simulink model "Q5_three_chart_system"  (R2024b)
settings: Solver=VariableStepAuto  StartTime=0.0  StopTime=100  RelTol=1e-3
model workspace (MAT data in the model file):
  K3 = 1
  M1 = 4
  M2 = 2
  M3 = 1
  b1 = 1
  b2 = 1
  b3 = 1
  k1 = 3
  k2 = 1
  k3 = 1
settings Model: Creator=chall  LastModifiedBy=chall

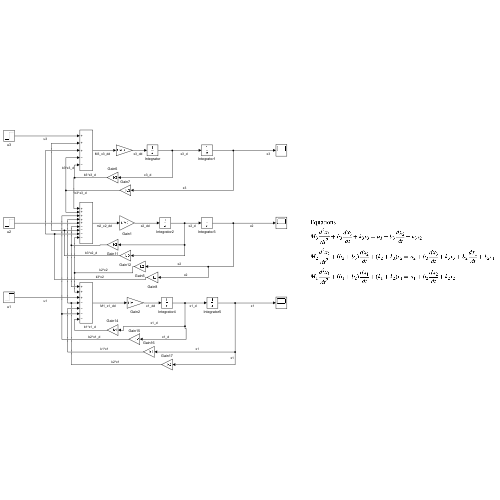
[thumbnail: Simulink's stored preview of the top-level diagram]
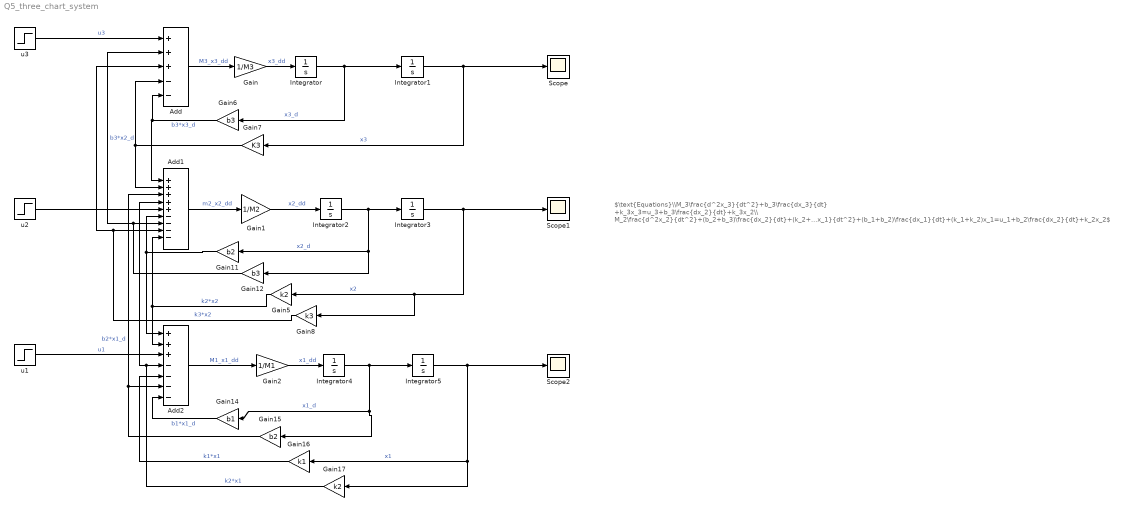
== system Q5_three_chart_system ==
  note: $\text{Equations}\\M_3\frac{d^2x_3}{dt^2}+b_3\frac{dx_3}{dt} +k_3x_3=u_3+b_3\frac{dx_2}{dt}+k_3x_2\\ M_2\frac{d^2x_2}{dt^2}+(b_2+b_3)\frac{dx_2}{dt}+(k_2+k_3)x_2=u_2+b_3\frac{dx_3}{dt}+k_3x_3+b_2\frac{dx_1}{dt}+k_2x_1\\M_1\frac{d^2x_1}{dt^2}+(b_1+b_2)\frac{dx_1}{dt}+(k_1+k_2)x_1=u_1+b_2\frac{dx_2}{dt}+k_2x_2$
  Add : Sum  Inputs=+++--
  Add1 : Sum  Inputs=+++++----
  Add2 : Sum  Inputs=+++----
  Gain : Gain  Gain=1/M3
  Gain1 : Gain  Gain=1/M2
  Gain11 : Gain  Gain=b2
  Gain12 : Gain  Gain=b3
  Gain14 : Gain  Gain=b1
  Gain15 : Gain  Gain=b2
  Gain16 : Gain  Gain=k1
  Gain17 : Gain  Gain=k2
  Gain2 : Gain  Gain=1/M1
  Gain5 : Gain  Gain=k2
  Gain6 : Gain  Gain=b3
  Gain7 : Gain  Gain=K3
  Gain8 : Gain  Gain=k3
  Integrator{,1..5} (6 alike) : Integrator
  Scope : Scope
  Scope1 : Scope
  Scope2 : Scope
  u1 : Step  Time=0  SampleTime=0
  u2 : Step  Time=0  SampleTime=0
  u3 : Step  Time=0  SampleTime=0
  wires:
  Add/1 -> Gain/1  "M3_x3_dd"
  Gain/1 -> Integrator/1  "x3_dd"
  Add1/1 -> Gain1/1  "m2_x2_dd"
  Gain1/1 -> Integrator2/1  "x2_dd"
  Integrator/1 -> Integrator1/1, Gain6/1  "x3_d"
  Integrator2/1 -> Gain11/1, Gain12/1, Integrator3/1  "x2_d"
  Integrator4/1 -> Integrator5/1, Gain15/1, Gain14/1  "x1_d"
  Gain2/1 -> Integrator4/1  "x1_dd"
  Integrator1/1 -> Scope/1, Gain7/1  "x3"
  Integrator3/1 -> Scope1/1, Gain8/1, Gain5/1  "x2"
  Integrator5/1 -> Scope2/1, Gain17/1, Gain16/1  "x1"
  Add2/1 -> Gain2/1  "M1_x1_dd"
  Gain6/1 -> Add1/1, Add/5  "b3*x3_d"
  Gain7/1 -> Add1/2, Add/4
  Gain15/1 -> Add1/3, Add2/6  "b2*x1_d"
  Gain17/1 -> Add2/4, Add1/4  "k2*x1"
  Gain11/1 -> Add2/1, Add1/6
  Gain12/1 -> Add/2, Add1/7  "b3*x2_d"
  Gain8/1 -> Add1/8, Add/3  "k3*x2"
  Gain5/1 -> Add1/9, Add2/2  "k2*x2"
  u1/1 -> Add2/3  "u1"
  u2/1 -> Add1/5
  u3/1 -> Add/1  "u3"
  Gain16/1 -> Add2/5  "k1*x1"
  Gain14/1 -> Add2/7  "b1*x1_d"
